simulink model "lab4teleia5"  (R2021a)
settings: Solver=ode23tb  StartTime=0.0  StopTime=10  MaxStep=1e-4  RelTol=1e-3
libraries: spsVoltageMeasurementLib x9, spsRMSLib x8, spsCurrentMeasurementLib x6, spsNeutralLib x3, spsACVoltageSourceLib x3, spsSeriesRLCBranchLib x3, spsMeanLib x2, simulink x2, spsDCVoltageSourceLib x1, spsThreePhaseSeriesRLCBranchLib x1, spsThreePhaseSeriesRLCLoadLib x1, spsPower3phInstantaneousLib x1
settings Model: Creator=User  LastModifiedBy=stama
settings SolverCC: AlgebraicLoopSolver=TrustRegion
settings DebuggingCC: SFMachineParentedDataDiag=warning  ArithmeticOperatorsInVariantConditions=warning
settings SFSimCC: CustomCodeUndefinedFunction=UseInterfaceOnly

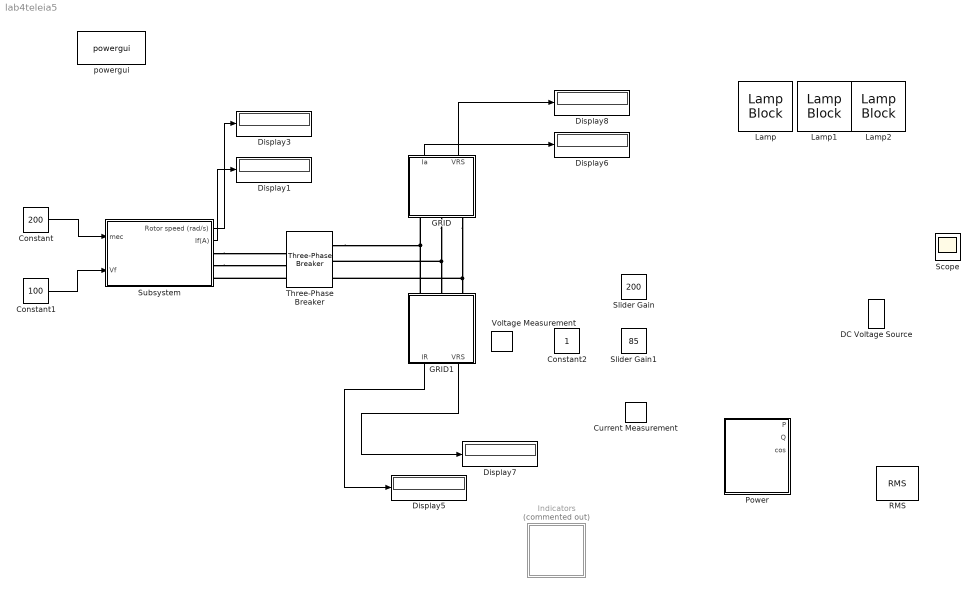
== system lab4teleia5 ==
  Constant : Constant  Value=200
  Constant1 : Constant  Value=100
  Constant2 : Constant
  Current Measurement : spsCurrentMeasurementLib/Current Measurement  PhasorSimulation=off  OutputType=Complex  PSBequivalent=0
  DC Voltage Source : spsDCVoltageSourceLib/DC Voltage Source  Amplitude=100  Measurements=None
  Display{1,3,5..8} (6 alike) : Display
  GRID : Subsystem
      mask DialogControl Label1 Prompt: Power Grid
  GRID1 : Subsystem
      mask DialogControl Label1 Prompt: Power Grid
  Indicators : Subsystem  Commented=on
      mask DialogControl Label1 Prompt: Indicator Lights
  Lamp : LampBlock  LabelPosition=Bottom
  Lamp1 : LampBlock  LabelPosition=Bottom
  Lamp2 : LampBlock  LabelPosition=Bottom
  Power : Subsystem
      mask DialogControl Control2 Prompt: Three phase power measurement
  RMS : spsRMSLib/RMS  TrueRMS=on  Freq=50  RMSInit=0  Ts=0
  Scope : Scope  NumInputPorts=2
  Slider Gain : simulink/Math Operations/Slider Gain  gain=200  low=1  high=10000
  Slider Gain1 : simulink/Math Operations/Slider Gain  gain=85  low=0  high=220
  Subsystem : Subsystem
      mask DialogControl Label1 Prompt: 8.1kVA, 400V, 4 poles
  Three-Phase Breaker : spsThreePhaseBreakerLib/Three-Phase Breaker  InitialState=open  SwitchA=on  SwitchB=on  SwitchC=on  SwitchTimes="[1/60  5/60]"  External=on  BreakerResistance=0.01  SnubberResistance=inf  SnubberCapacitance=inf  Measurements=None
  Voltage Measurement : spsVoltageMeasurementLib/Voltage Measurement  PhasorSimulation=off  OutputType=Complex  PSBequivalent=0
  powergui : spspowerguiLib/powergui  Priority=1  SimulationMode=Continuous  SampleTime=50e-6  frequency=60  Iterations=50  frequencyindice=50  Pbase=100e6  ErrMax=1e-4  UnitsV=kV  UnitsW=MW  buscounter=0  FunctionMessages=off  echomessages=off  EnableUseOfTLC=off  CurrentSourceSwitches=off  DisableSnubberDevices=off  DisableRonSwitches=off  DisableVfSwitches=off  DisplayEquations=off  AutomaticDiscreteSolvers=off  SolverType=Tustin/Backward Euler (TBE)  Interpol=off  ExternalGateDelay=off  methode=off  Ts=100  x0status=blocks  SPID=on  SwTol=0  HookPort=off  NonlinearTolerance=1e-4  nMaxIteration=100  ContinueOnMaxIteration=off  RestoreLinks=warning  ResistiveCurrentMeasurement=off  Frange=[0:2:500]  Ylog=off  Xlog=on  ShowGrid=off  save=off  variable=ZData  structure=0  ZoomFFT=off  StartTime=0.0  cycles=1  DisplayStyle=1  fundamental=60  FreqAxis=off  MaxFrequency=1000  frequencyindicesteady=1  RmsSteady=1  display=off
  wires:
  GRID1/1(IR) -> Display5/1
  GRID/1(Ia) -> Display6/1
  GRID1/2(VRS) -> Display7/1
  GRID/2(VRS) -> Display8/1
  Constant1/1 -> Subsystem/2(Vf)
  Constant/1 -> Subsystem/1(mec)
  Subsystem/1(Rotor speed (rad/s)) -> Display3/1
  Subsystem/2(Ιf(A)) -> Display1/1
  connections:
  GRID1/LConn1 -- GRID/LConn1 -- Three-Phase Breaker/RConn1
  GRID/LConn2 -- Three-Phase Breaker/RConn2 -- GRID1/LConn2
  GRID/LConn3 -- Three-Phase Breaker/RConn3 -- GRID1/LConn3
  Subsystem/RConn1 -- Three-Phase Breaker/LConn1
  Subsystem/RConn2 -- Three-Phase Breaker/LConn2
  Three-Phase Breaker/LConn3 -- Subsystem/RConn3

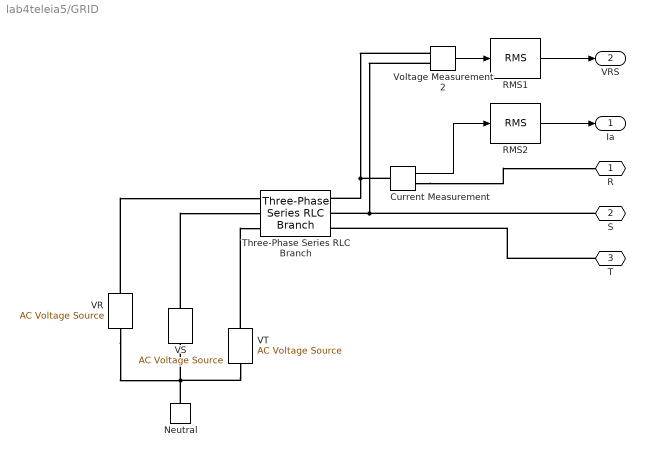
== system lab4teleia5/GRID ==
  Current Measurement : spsCurrentMeasurementLib/Current Measurement  PhasorSimulation=off  OutputType=Complex  PSBequivalent=0
  Neutral : spsNeutralLib/Neutral  LConnTagsString=a  NodeNumber=10
      settings: AttributesFormatString=node %<NodeNumber>  SourceProductBaseCode=PS
  RMS1 : spsRMSLib/RMS  TrueRMS=on  Freq=50  RMSInit=0  Ts=0
  RMS2 : spsRMSLib/RMS  TrueRMS=on  Freq=50  RMSInit=0  Ts=0
  Three-Phase Series RLC Branch : spsThreePhaseSeriesRLCBranchLib/Three-Phase Series RLC Branch  LConnTagsString=A|B|C  RConnTagsString=A|B|C  BranchType=RL  Resistance=1e-3  Inductance=1e-5  Capacitance=1e-6  Measurements=None
  VR : spsACVoltageSourceLib/AC Voltage Source  Amplitude=325.27  Phase=0  Frequency=50  SampleTime=0  Measurements=None  BusType=swing  Pref=10e3  Qref=0  Qmin=-inf  Qmax=+inf
  VS : spsACVoltageSourceLib/AC Voltage Source  Amplitude=325.27  Phase=-120  Frequency=50  SampleTime=0  Measurements=None  BusType=swing  Pref=10e3  Qref=0  Qmin=-inf  Qmax=+inf
  VT : spsACVoltageSourceLib/AC Voltage Source  Amplitude=325.27  Phase=120  Frequency=50  SampleTime=0  Measurements=None  BusType=swing  Pref=10e3  Qref=0  Qmin=-inf  Qmax=+inf
  Voltage Measurement2 : spsVoltageMeasurementLib/Voltage Measurement  PhasorSimulation=off  OutputType=Complex  PSBequivalent=0
  R : PMIOPort  Side=Left
  S : PMIOPort  Port=2  Side=Left
  T : PMIOPort  Port=3  Side=Left
  Ia : Outport
  VRS : Outport  Port=2
  wires:
  RMS2/1 -> Ia/1
  Current Measurement/1 -> RMS2/1
  RMS1/1 -> VRS/1
  Voltage Measurement2/1 -> RMS1/1
  connections:
  Neutral/LConn1 -- VS/LConn1 -- VT/LConn1 -- VR/LConn1
  S/RConn1 -- Voltage Measurement2/LConn2 -- Three-Phase Series RLC Branch/RConn2
  T/RConn1 -- Three-Phase Series RLC Branch/RConn3
  VR/RConn1 -- Three-Phase Series RLC Branch/LConn1
  VS/RConn1 -- Three-Phase Series RLC Branch/LConn2
  VT/RConn1 -- Three-Phase Series RLC Branch/LConn3
  Current Measurement/LConn1 -- Voltage Measurement2/LConn1 -- Three-Phase Series RLC Branch/RConn1
  Current Measurement/RConn1 -- R/RConn1

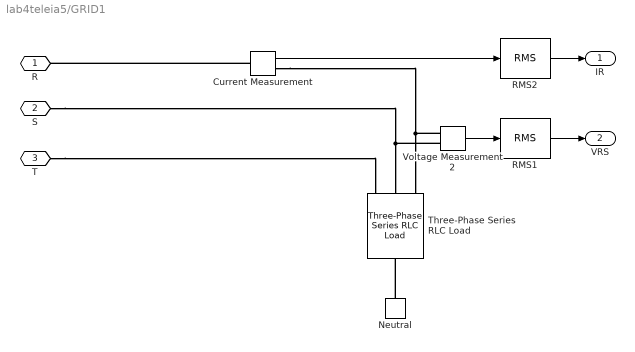
== system lab4teleia5/GRID1 ==
  Current Measurement : spsCurrentMeasurementLib/Current Measurement  PhasorSimulation=off  OutputType=Complex  PSBequivalent=0
  Neutral : spsNeutralLib/Neutral  LConnTagsString=a  NodeNumber=10
      settings: AttributesFormatString=node %<NodeNumber>  SourceProductBaseCode=PS
  RMS1 : spsRMSLib/RMS  TrueRMS=on  Freq=50  RMSInit=0  Ts=0
  RMS2 : spsRMSLib/RMS  TrueRMS=on  Freq=50  RMSInit=0  Ts=0
  Three-Phase Series RLC Load : spsThreePhaseSeriesRLCLoadLib/Three-Phase Series RLC Load  LConnTagsString=A|B|C  RConnTagsString=N  Configuration=Y (neutral)  NominalVoltage=400  Vabc=[1e3 1e3 1e3]  Vabcp=[1e3 1e3 1e3]  NominalFrequency=50  UnbalancedPower=off  ActivePower=1e4  InductivePower=1000  CapacitivePower=0  Pabc=[10e3 9e3 11e3]  QLabc=[100 90 110]  QCabc=[100 90 110]  Pabcp=[10e3 9e3 11e3]  QLabcp=[100 90 110]  QCabcp=[100 90 110]  Measurements=None  LoadType=constant Z
  Voltage Measurement2 : spsVoltageMeasurementLib/Voltage Measurement  PhasorSimulation=off  OutputType=Complex  PSBequivalent=0
  R : PMIOPort  Side=Left
  S : PMIOPort  Port=2  Side=Left
  T : PMIOPort  Port=3  Side=Left
  IR : Outport
  VRS : Outport  Port=2
  wires:
  Current Measurement/1 -> RMS2/1
  RMS2/1 -> IR/1
  Voltage Measurement2/1 -> RMS1/1
  RMS1/1 -> VRS/1
  connections:
  S/RConn1 -- Voltage Measurement2/LConn2 -- Three-Phase Series RLC Load/LConn2
  T/RConn1 -- Three-Phase Series RLC Load/LConn1
  Current Measurement/RConn1 -- Voltage Measurement2/LConn1 -- Three-Phase Series RLC Load/LConn3
  Current Measurement/LConn1 -- R/RConn1
  Neutral/LConn1 -- Three-Phase Series RLC Load/RConn1

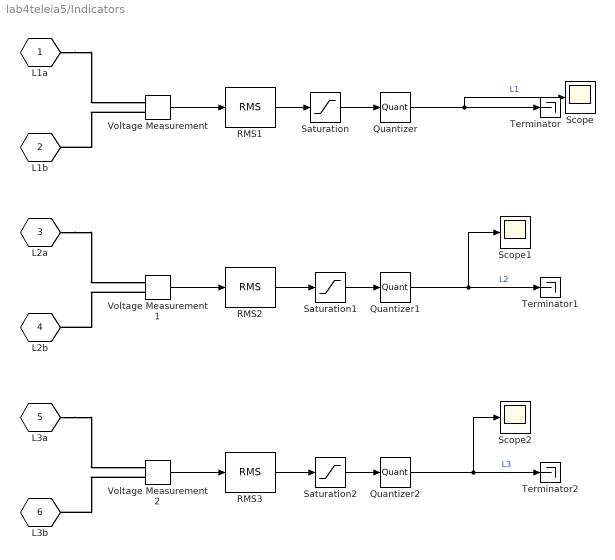
== system lab4teleia5/Indicators ==
  Quantizer : Quantizer  QuantizationInterval=20
  Quantizer1 : Quantizer  QuantizationInterval=20
  Quantizer2 : Quantizer  QuantizationInterval=20
  RMS1 : spsRMSLib/RMS  TrueRMS=on  Freq=50  RMSInit=0  Ts=0
  RMS2 : spsRMSLib/RMS  TrueRMS=on  Freq=50  RMSInit=0  Ts=0
  RMS3 : spsRMSLib/RMS  TrueRMS=on  Freq=50  RMSInit=0  Ts=0
  Saturation : Saturate  UpperLimit=60  LowerLimit=0
  Saturation1 : Saturate  UpperLimit=60  LowerLimit=0
  Saturation2 : Saturate  UpperLimit=60  LowerLimit=0
  Scope : Scope
  Scope1 : Scope
  Scope2 : Scope
  Terminator : Terminator
  Terminator1 : Terminator
  Terminator2 : Terminator
  Voltage Measurement : spsVoltageMeasurementLib/Voltage Measurement  PhasorSimulation=off  OutputType=Complex  PSBequivalent=0
  Voltage Measurement1 : spsVoltageMeasurementLib/Voltage Measurement  PhasorSimulation=off  OutputType=Complex  PSBequivalent=0
  Voltage Measurement2 : spsVoltageMeasurementLib/Voltage Measurement  PhasorSimulation=off  OutputType=Complex  PSBequivalent=0
  L1a : PMIOPort  Tag=PMCPort  Side=Left
  L1b : PMIOPort  Tag=PMCPort  Port=2  Side=Right
  L2a : PMIOPort  Tag=PMCPort  Port=3  Side=Left
  L2b : PMIOPort  Tag=PMCPort  Port=4  Side=Right
  L3a : PMIOPort  Tag=PMCPort  Port=5  Side=Left
  L3b : PMIOPort  Tag=PMCPort  Port=6  Side=Right
  wires:
  Voltage Measurement/1 -> RMS1/1
  Quantizer/1 -> Scope/1, Terminator/1  "L1"
  Quantizer1/1 -> Scope1/1, Terminator1/1  "L2"
  Voltage Measurement1/1 -> RMS2/1
  Voltage Measurement2/1 -> RMS3/1
  RMS2/1 -> Saturation1/1
  RMS1/1 -> Saturation/1
  RMS3/1 -> Saturation2/1
  Quantizer2/1 -> Scope2/1, Terminator2/1  "L3"
  Saturation/1 -> Quantizer/1
  Saturation1/1 -> Quantizer1/1
  Saturation2/1 -> Quantizer2/1
  connections:
  L1a/RConn1 -- Voltage Measurement/LConn1
  Voltage Measurement/LConn2 -- L1b/RConn1
  L2a/RConn1 -- Voltage Measurement1/LConn1
  Voltage Measurement1/LConn2 -- L2b/RConn1
  L3a/RConn1 -- Voltage Measurement2/LConn1
  Voltage Measurement2/LConn2 -- L3b/RConn1

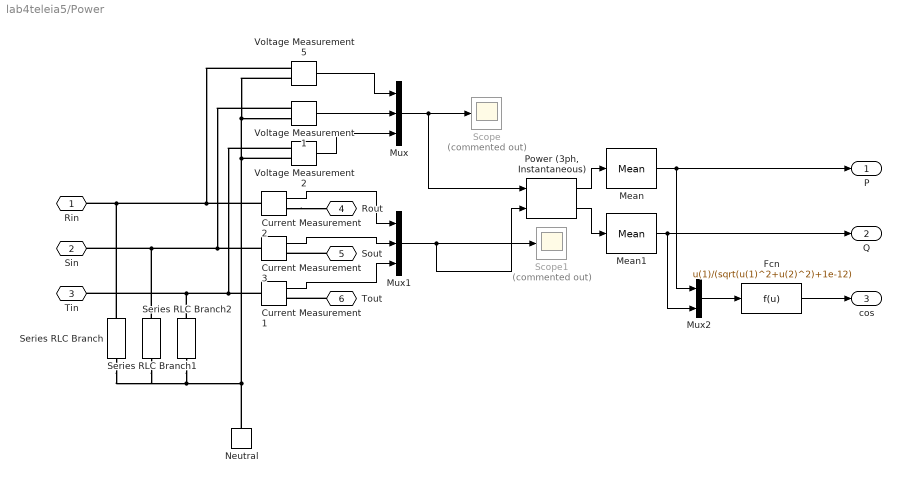
== system lab4teleia5/Power ==
  Current Measurement1 : spsCurrentMeasurementLib/Current Measurement  PhasorSimulation=off  OutputType=Complex  PSBequivalent=0
  Current Measurement2 : spsCurrentMeasurementLib/Current Measurement  PhasorSimulation=off  OutputType=Complex  PSBequivalent=0
  Current Measurement3 : spsCurrentMeasurementLib/Current Measurement  PhasorSimulation=off  OutputType=Complex  PSBequivalent=0
  Fcn : Fcn  Expr=u(1)/(sqrt(u(1)^2+u(2)^2)+1e-12)
  Mean : spsMeanLib/Mean  Freq=50  Vinit=0  Ts=0
  Mean1 : spsMeanLib/Mean  Freq=50  Vinit=0  Ts=0
  Mux : Mux  Inputs=3
  Mux1 : Mux  Inputs=3
  Mux2 : Mux  Inputs=2
  Neutral : spsNeutralLib/Neutral  LConnTagsString=a  NodeNumber=10
      settings: AttributesFormatString=node %<NodeNumber>  SourceProductBaseCode=PS
  "Power (3ph, Instantaneous)" : spsPower3phInstantaneousLib/Power (3ph, Instantaneous)
  Scope : Scope  Commented=on
  Scope1 : Scope  Commented=on
  Series RLC Branch : spsSeriesRLCBranchLib/Series RLC Branch  LConnTagsString=__new0  RConnTagsString=__new0  BranchType=R  Resistance=1e6  Inductance=1e-3  SetiL0=off  InitialCurrent=0  Capacitance=1e-6  Setx0=off  InitialVoltage=0  Measurements=None
  Series RLC Branch1 : spsSeriesRLCBranchLib/Series RLC Branch  LConnTagsString=__new0  RConnTagsString=__new0  BranchType=R  Resistance=1e6  Inductance=1e-3  SetiL0=off  InitialCurrent=0  Capacitance=1e-6  Setx0=off  InitialVoltage=0  Measurements=None
  Series RLC Branch2 : spsSeriesRLCBranchLib/Series RLC Branch  LConnTagsString=__new0  RConnTagsString=__new0  BranchType=R  Resistance=1e6  Inductance=1e-3  SetiL0=off  InitialCurrent=0  Capacitance=1e-6  Setx0=off  InitialVoltage=0  Measurements=None
  Voltage Measurement1 : spsVoltageMeasurementLib/Voltage Measurement  PhasorSimulation=off  OutputType=Complex  PSBequivalent=0
  Voltage Measurement2 : spsVoltageMeasurementLib/Voltage Measurement  PhasorSimulation=off  OutputType=Complex  PSBequivalent=0
  Voltage Measurement5 : spsVoltageMeasurementLib/Voltage Measurement  PhasorSimulation=off  OutputType=Complex  PSBequivalent=0
  Rin : PMIOPort  Side=Left
  Sin : PMIOPort  Port=2  Side=Left
  Tin : PMIOPort  Port=3  Side=Left
  Rout : PMIOPort  Port=4  Side=Right
  Sout : PMIOPort  Port=5  Side=Right
  Tout : PMIOPort  Port=6  Side=Right
  P : Outport
  Q : Outport  Port=2
  cos : Outport  Port=3
  wires:
  "Power (3ph, Instantaneous)"/1 -> Mean/1
  Mux/1 -> "Power (3ph, Instantaneous)"/1, Scope/1
  Voltage Measurement5/1 -> Mux/1
  Voltage Measurement1/1 -> Mux/2
  Voltage Measurement2/1 -> Mux/3
  Current Measurement3/1 -> Mux1/2
  Current Measurement2/1 -> Mux1/1
  Current Measurement1/1 -> Mux1/3
  "Power (3ph, Instantaneous)"/2 -> Mean1/1
  Mean/1 -> Mux2/1, P/1
  Mux2/1 -> Fcn/1
  Fcn/1 -> cos/1
  Mean1/1 -> Mux2/2, Q/1
  Mux1/1 -> Scope1/1, "Power (3ph, Instantaneous)"/2
  connections:
  Current Measurement1/LConn1 -- Voltage Measurement2/LConn1 -- Series RLC Branch2/LConn1 -- Tin/RConn1
  Current Measurement3/LConn1 -- Voltage Measurement1/LConn1 -- Series RLC Branch1/LConn1 -- Sin/RConn1
  Current Measurement2/LConn1 -- Voltage Measurement5/LConn1 -- Series RLC Branch/LConn1 -- Rin/RConn1
  Voltage Measurement5/LConn2 -- Series RLC Branch/RConn1 -- Series RLC Branch1/RConn1 -- Series RLC Branch2/RConn1 -- Neutral/LConn1 -- Voltage Measurement2/LConn2 -- Voltage Measurement1/LConn2
  Current Measurement2/RConn1 -- Rout/RConn1
  Sout/RConn1 -- Current Measurement3/RConn1
  Tout/RConn1 -- Current Measurement1/RConn1

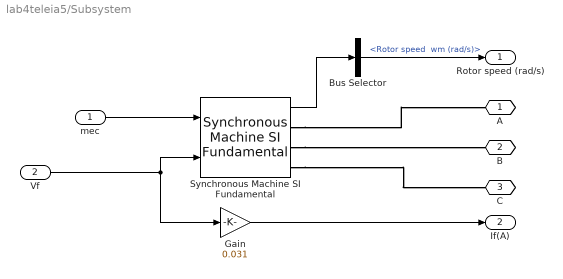
== system lab4teleia5/Subsystem ==
  mec : Inport
  Vf : Inport  Port=2
  Bus Selector : BusSelector  OutputSignals="Mechanical.Rotor speed  wm (rad/s)"
  Gain : Gain  Gain=0.031
  Synchronous Machine SI Fundamental : spsSynchronousMachineSIFundamentalLib/Synchronous Machine SI Fundamental  PresetModel=No  MechanicalLoad=Mechanical power Pm  ShowDetailedParameters=on  RotorType=Salient-pole  Units=SI fundamental parameters  MeasurementBus=off  NominalParameters=[8100 400 50 7]  Stator=[1.62 0.004527 0.1086 0.05175]  Field=[1.208 0.01132]  Dampers2=[ 0.0664, 1.387e-3, 0.0292, 6.896e-4, 7.907e-3, 2.477e-3]  Dampers1=[3.142 0.007334 4.772 0.01015]  Mechanical=[0.0923 0.009 2]  PolePairs=2  InitialConditions="[ 0  0  0  0  0  0  0  0  1]"  SetSaturation=on  Saturation=[695.64,774.7,917.5,1001.6,1082.2,1175.9,1293.6,1430.2,1583.7;9660,10623,12243,13063,13757,14437,15180,15890,16567]  DisplayVfd=off  LoadFlowParameters=[1,0,0,0,0]  TsPowergui=0  TsBlock=-1  IterativeModel=Trapezoidal non iterative  IterativeDiscreteModel=Trapezoidal non iterative  BusType=PV  Pref=0  Qref=0  Qmin=-inf  Qmax=inf  PLF=0  QLF=0
      settings: SourceProductBaseCode=PS
  A : PMIOPort  Side=Right
  B : PMIOPort  Port=2  Side=Right
  C : PMIOPort  Port=3  Side=Right
  Rotor speed (rad/s) : Outport
  Ιf(A) : Outport  Port=2
  wires:
  Synchronous Machine SI Fundamental/1 -> Bus Selector/1
  mec/1 -> Synchronous Machine SI Fundamental/1
  Bus Selector/1 -> Rotor speed (rad/s)/1  "<Rotor speed  wm (rad/s)>"
  Vf/1 -> Gain/1, Synchronous Machine SI Fundamental/2
  Gain/1 -> Ιf(A)/1
  connections:
  Synchronous Machine SI Fundamental/RConn2 -- B/RConn1
  Synchronous Machine SI Fundamental/RConn1 -- A/RConn1
  Synchronous Machine SI Fundamental/RConn3 -- C/RConn1
